simulink model "MPC_Quad"  (R2022b)
settings: Solver=FixedStepAuto  StartTime=0.0  StopTime=T_total  FixedStep=Ts  RelTol=1e-3
undefined symbols (not defined in the file): Alt_D, Alt_I, Alt_P, Att_Ang_P, Att_AngVel_D, Att_AngVel_I, Att_AngVel_P, Cm, Ct, DiscIntNeverNeededParam, estim_hover_nrpm, g, Ir, Ixx, Iyy, Izz, Length, mass, Pos_Pos_P, Pos_Vel_I, Pos_Vel_P, SampleTime, Yaw_D, Yaw_I, Yaw_P
libraries: slpidlib x4, simulink x2, mpclib x1
settings Model: PacingRate=0.350000  Creator=Bw Jiang  LastModifiedBy=Bw Jiang
settings DebuggingCC: AlgebraicLoopMsg=none  ParameterOverflowMsg=none  ParameterUnderflowMsg=error

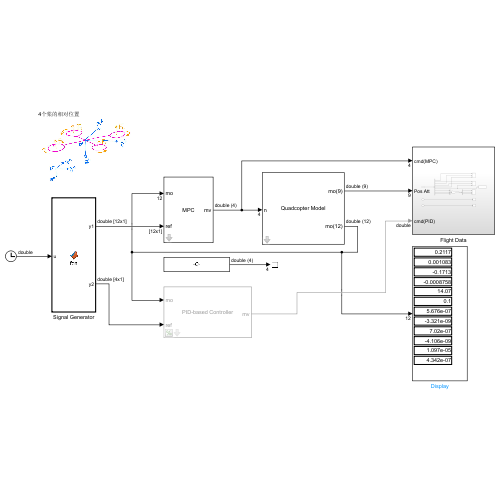
[thumbnail: Simulink's stored preview of the top-level diagram]
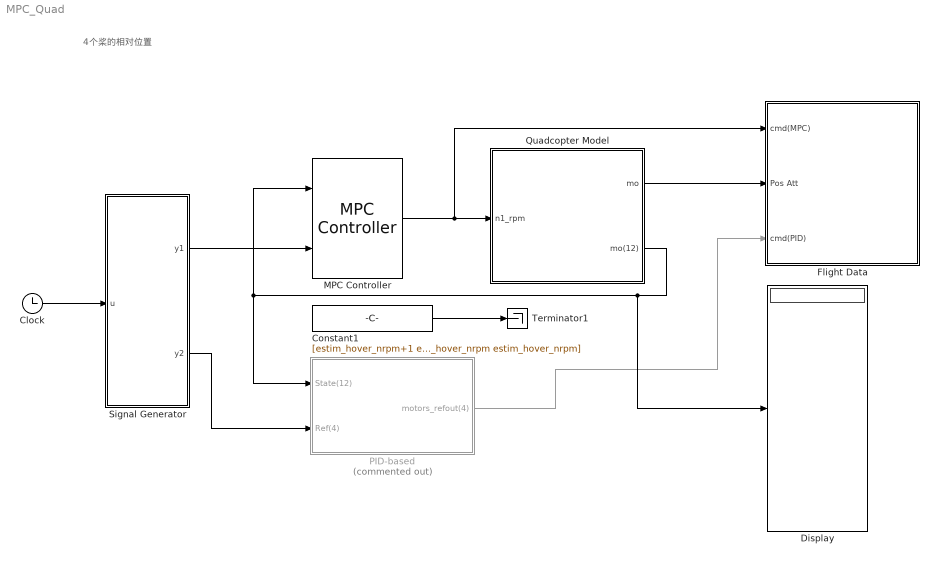
== system MPC_Quad ==
  note: 4个桨的相对位置
  Clock : Clock
  Constant1 : Constant  Value=[estim_hover_nrpm+1 estim_hover_nrpm estim_hover_nrpm estim_hover_nrpm]
  Display : Display
  Flight Data : Subsystem
  MPC Controller : mpclib/MPC Controller  SCDEnableBlockLinearizationSpecification=on  mpcobj=mpc1  is_multiple=0  enable_value=0  return_u0=off  updateMPCinCallerWorkspace=on  md_inport=off  mv_inport=off  uref_inport=off  return_cost=off  return_mvseq=off  return_qpstatus=off  return_xseq=off  return_state=off  return_ovseq=off  state_inport=off  umin_inport=off  umax_inport=off  ymin_inport=off  ymax_inport=off  cc_inport=off  ywt_inport=off  uwt_inport=off  duwt_inport=off  rhoeps_inport=off  pm_inport=off  MaximumP=10  HorizonChoice=FixedHorizon  n_ts=0.01  n_p=50  n_mv=4  n_md=0  n_ud=0  n_mo=12  n_uo=0  BlockDataType=double  SampleTimeInherited=off  switch_inport=off
  PID-based : Subsystem  Commented=on  mask{SampleTime=SampleTime, Pos_Pos_P=Pos_Pos_P, Pos_Vel_P=Pos_Vel_P, Pos_Vel_I=Pos_Vel_I, Alt_P=Alt_P, Alt_I=Alt_I, Alt_D=Alt_D, Yaw_P=Yaw_P, Yaw_I=Yaw_I, Yaw_D=Yaw_D, Att_Ang_P=Att_Ang_P, Att_AngVel_P=Att_AngVel_P, Att_AngVel_I=Att_AngVel_I, Att_AngVel_D=Att_AngVel_D}
      mask prompts: Pos_Pos_P "PosController.PositionLoop.P"; Pos_Vel_P "PosController.VelocityLoop.P"; Pos_Vel_I "PosController.VelocityLoop.I"; Alt_P "AltController.P"; Alt_I "AltController.I"; Alt_D "AltController.D"; Yaw_P "YawController.P"; Yaw_I "YawController.I"; Yaw_D "YawController.D"; Att_Ang_P "AttController.AngleLoop.P"; Att_AngVel_P "AttController.AngleVelocityLoop.P"; Att_AngVel_I "AttController.AngleVelocityLoop.I"; Att_AngVel_D "AttController.AngleVelocityLoop.D"
      mask init:
      | run("Scripts\PID_based_controller_init.m");
      mask DialogControl ParameterGroupVar Prompt: 参数
      mask Display:
      | disp('PID-based Controller');
      | port_label('output', 1, 'mv')
      | port_label('input', 1, 'mo')
      | port_label('input', 2, 'ref')
  Quadcopter Model : Subsystem  mask{g=g, mass=mass, I_xx=Ixx, I_yy=Iyy, I_zz=Izz, I_r=Ir, L=Length, C_M=Cm, C_T=Ct}
      mask prompts: g "Gravity"; I_xx "Inertia_xx"; I_yy "Inertia_yy"; I_zz "Inertia_zz"; I_r "Inertia_per_rotor"; L "Length"
      mask DialogControl ParameterGroupVar Prompt: 参数
      mask Display:
      | disp('Quadcopter Model');
      | port_label('input', 1, 'n')
      | % port_label('input', 2, 'n2')
      | % port_label('input', 3, 'n3')
      | % port_label('input', 4, 'n4')
      | port_label('output', 1, 'mo(9)')
      | port_label('output', 2, 'mo(12)')
      | % port_label('output', 3, 'y')
      | % port_label('output', 4, 'vy')
      | % port_label('output', 5, 'z')
      | % port_label('output', 6, 'vz')
      | % port_label('output', 7, 'phi')
      | % port_label('output', 8, 'd_phi')
      | % port_label('output', 9, 'theta')
      | % port_label('output', 10, 'd_theta')
      | % port_label('output', 11, 'psi')
      | % port_label('output', 12, 'd_psi')
  Signal Generator : MATLAB Function  TreatAsAtomicUnit=on
  Terminator1 : Terminator
  wires:
  Signal Generator/1(y1) -> MPC Controller/2
  Clock/1 -> Signal Generator/1(u)
  PID-based/1(motors_refout(4)) -> Flight Data/3(cmd(PID))
  MPC Controller/1 -> Quadcopter Model/1(n1_rpm), Flight Data/1(cmd(MPC))
  Signal Generator/2(y2) -> PID-based/2(Ref(4))
  Constant1/1 -> Terminator1/1
  Quadcopter Model/1(mo) -> Flight Data/2(Pos Att)
  Quadcopter Model/2(mo(12)) -> Display/1, MPC Controller/1, PID-based/1(State(12))

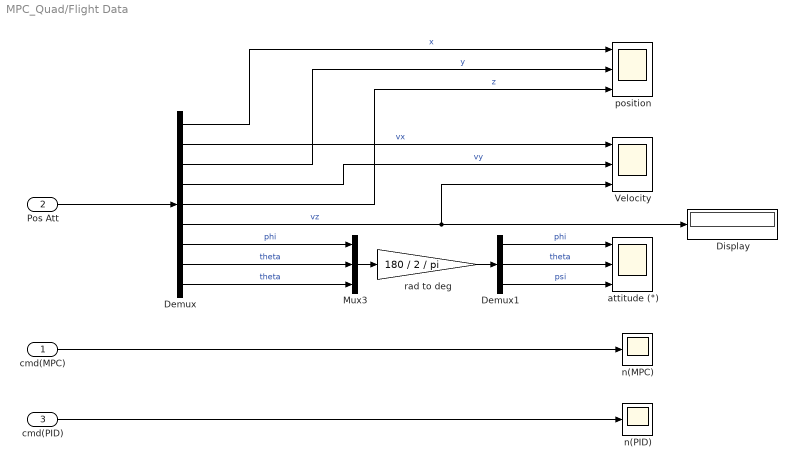
== system MPC_Quad/Flight Data ==
  cmd(MPC) : Inport
  Pos Att : Inport  Port=2
  cmd(PID) : Inport  Port=3
  Demux : Demux  Outputs=9
  Demux1 : Demux  Outputs=3
  Display : Display
  Mux3 : Mux  Inputs=3
  Velocity : Scope  NumInputPorts=3
  attitude (°) : Scope  NumInputPorts=3
  n(MPC) : Scope
  n(PID) : Scope
  position : Scope  NumInputPorts=3
  rad to deg : Gain  Gain=180 / 2 / pi
  wires:
  Demux/8 -> Mux3/2  "theta"
  Demux/4 -> Velocity/2  "vy"
  Demux/2 -> Velocity/1  "vx"
  Demux/7 -> Mux3/1  "phi"
  Demux/6 -> Velocity/3, Display/1  "vz"
  cmd(PID)/1 -> n(PID)/1
  Demux/5 -> position/3  "z"
  Demux/1 -> position/1  "x"
  Demux1/1 -> attitude (°)/1  "phi"
  Demux/3 -> position/2  "y"
  Demux1/2 -> attitude (°)/2  "theta"
  rad to deg/1 -> Demux1/1
  Demux1/3 -> attitude (°)/3  "psi"
  Mux3/1 -> rad to deg/1
  cmd(MPC)/1 -> n(MPC)/1
  Pos Att/1 -> Demux/1
  Demux/9 -> Mux3/3  "theta"

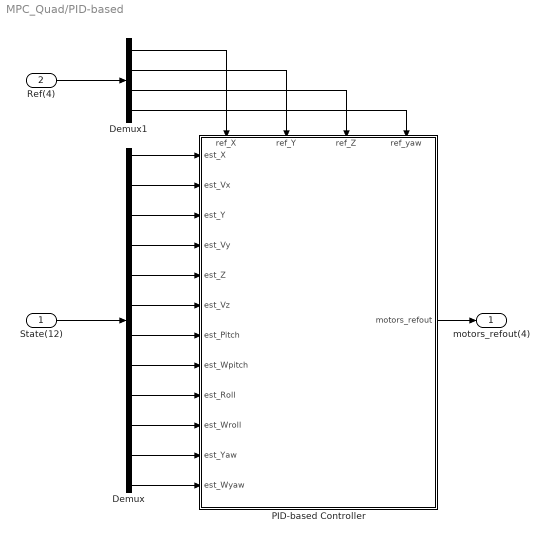
== system MPC_Quad/PID-based ==
  State(12) : Inport
  Ref(4) : Inport  Port=2
  Demux : Demux  Outputs=12
  Demux1 : Demux
  PID-based Controller : Subsystem
      settings: PortSchema="{\"entries\":[{\"content\":{\"sides\":[{\"content\":{\"connectorIds\":[\"In1\",\"In2\",\"In3\",\"In4\",\"In5\",\"In6\",\"In7\",\"In8\",\"In9\",\"In10\",\"In11\",\"In12\"]},\"type\":\"ConnectorPlacement.EquallySpacedRectSide\",\"uuid\":\"809a58d1-8f24-4346-a9a1-bdf3f40071a9\"},{\"content\":{\"connectorIds\":[\"Out1\"],\"side\":\"RIGHT\"},\"type\":\"ConnectorPlacement.EquallySpacedRectSide\",\"uuid\":\"e36db7a5-8644-49ff-9b48-8e381d81be19\"},{\"content\":{\"connectorIds\":[\"In13\",\"In14\",\"In15\",\"In16\"],\"side\":\"TOP\"},\"type\":\"ConnectorPlacement.EquallySpacedRectSide\",\"uuid\":\"d8c211b6-7652-4be5-9d63-16c6c31a5cb3\"}]},\"type\":\"ConnectorPlacement.EquallySpacedConnector\",\"uuid\":\"28a38415-8484-4982-8141-ea2d794bbc37\"}],\"packageUris\":[\"http://schema.mathworks.com/mf0/Connector/R2020b\"],\"version\":\"1.0\"}"
  motors_refout(4) : Outport
  wires:
  State(12)/1 -> Demux/1
  Demux1/1 -> PID-based Controller/13(ref_X)
  Demux1/2 -> PID-based Controller/14(ref_Y)
  Demux/5 -> PID-based Controller/5(est_Z)
  Demux/6 -> PID-based Controller/6(est_Vz)
  Demux/12 -> PID-based Controller/12(est_Wyaw)
  Demux/2 -> PID-based Controller/2(est_Vx)
  Demux1/3 -> PID-based Controller/15(ref_Z)
  Demux/11 -> PID-based Controller/11(est_Yaw)
  Demux/1 -> PID-based Controller/1(est_X)
  Demux/3 -> PID-based Controller/3(est_Y)
  Demux/4 -> PID-based Controller/4(est_Vy)
  Demux1/4 -> PID-based Controller/16(ref_yaw)
  PID-based Controller/1(motors_refout) -> motors_refout(4)/1
  Ref(4)/1 -> Demux1/1
  Demux/7 -> PID-based Controller/7(est_Pitch)
  Demux/8 -> PID-based Controller/8(est_Wpitch)
  Demux/9 -> PID-based Controller/9(est_Roll)
  Demux/10 -> PID-based Controller/10(est_Wroll)

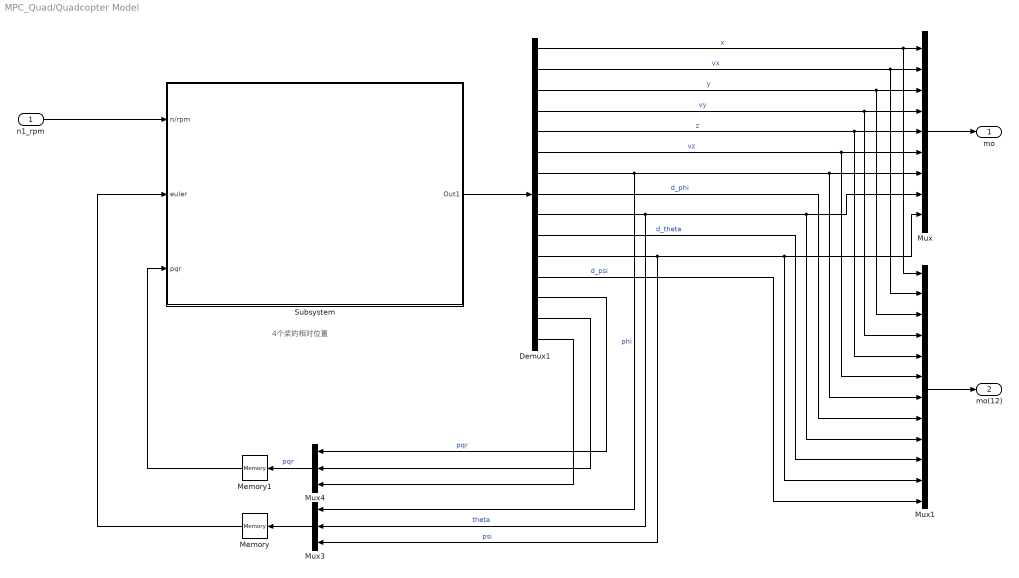
== system MPC_Quad/Quadcopter Model ==
  note: 4个桨的相对位置
  n1_rpm : Inport
  Demux1 : Demux  Outputs=15
  Memory : Memory  InheritSampleTime=on
  Memory1 : Memory  InheritSampleTime=on
  Mux : Mux  Inputs=9
  Mux1 : Mux  Inputs=12
  Mux3 : Mux  Inputs=3
  Mux4 : Mux  Inputs=3
  Subsystem : Subsystem
  mo : Outport
  mo(12) : Outport  Port=2
  wires:
  n1_rpm/1 -> Subsystem/1(n/rpm)
  Mux/1 -> mo/1
  Mux1/1 -> mo(12)/1
  Memory1/1 -> Subsystem/3(pqr)
  Demux1/15 -> Mux4/3
  Demux1/8 -> Mux1/8  "d_phi"
  Demux1/13 -> Mux4/1  "pqr"
  Mux4/1 -> Memory1/1  "pqr"
  Demux1/9 -> Mux/8, Mux1/9, Mux3/2  "theta"
  Demux1/10 -> Mux1/10  "d_theta"
  Demux1/1 -> Mux1/1, Mux/1  "x"
  Demux1/2 -> Mux/2, Mux1/2  "vx"
  Demux1/11 -> Mux/9, Mux1/11, Mux3/3  "psi"
  Demux1/4 -> Mux/4, Mux1/4  "vy"
  Demux1/3 -> Mux/3, Mux1/3  "y"
  Demux1/5 -> Mux/5, Mux1/5  "z"
  Subsystem/1(Out1) -> Demux1/1
  Demux1/12 -> Mux1/12  "d_psi"
  Memory/1 -> Subsystem/2(euler)
  Demux1/6 -> Mux/6, Mux1/6  "vz"
  Demux1/7 -> Mux/7, Mux1/7, Mux3/1  "phi"
  Mux3/1 -> Memory/1
  Demux1/14 -> Mux4/2

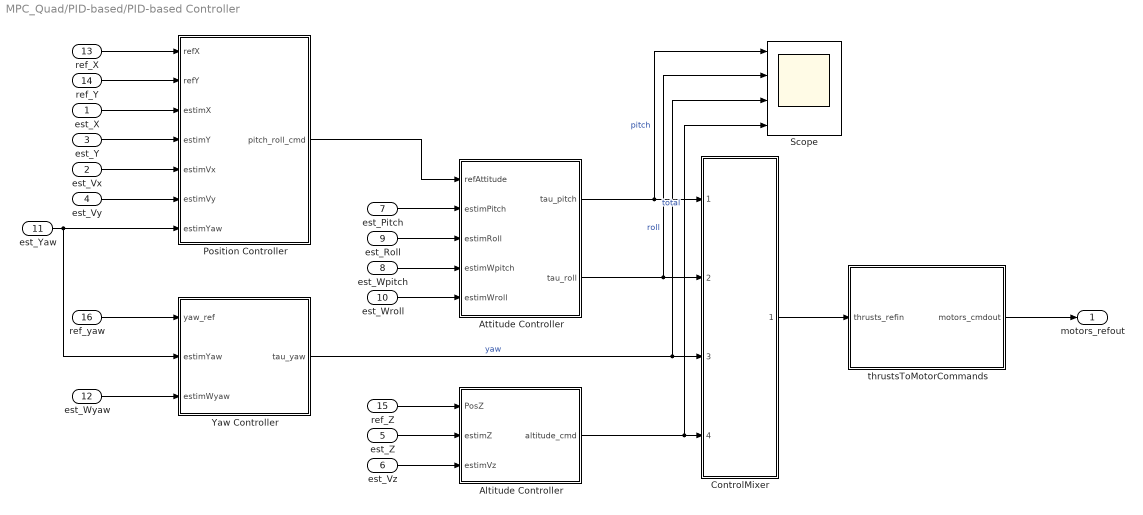
== system MPC_Quad/PID-based/PID-based Controller ==
  est_X : Inport
  est_Vx : Inport  Port=2
  est_Y : Inport  Port=3
  est_Vy : Inport  Port=4
  est_Z : Inport  Port=5
  est_Vz : Inport  Port=6
  est_Pitch : Inport  Port=7
  est_Wpitch : Inport  Port=8
  est_Roll : Inport  Port=9
  est_Wroll : Inport  Port=10
  est_Yaw : Inport  Port=11
  est_Wyaw : Inport  Port=12
  ref_X : Inport  Port=13
  ref_Y : Inport  Port=14
  ref_Z : Inport  Port=15
  ref_yaw : Inport  Port=16
  Altitude Controller : Subsystem
  Attitude Controller : Subsystem
  ControlMixer : Subsystem
  Position Controller : Subsystem
  Scope : Scope  NumInputPorts=4
  Yaw Controller : Subsystem
  thrustsToMotorCommands : Subsystem
  motors_refout : Outport  VectorParamsAs1DForOutWhenUnconnected=off
  wires:
  ControlMixer/1(thrusts_refout) -> thrustsToMotorCommands/1(thrusts_refin)
  est_X/1 -> Position Controller/3(estimX)
  est_Pitch/1 -> Attitude Controller/2(estimPitch)
  est_Vz/1 -> Altitude Controller/3(estimVz)
  ref_X/1 -> Position Controller/1(refX)
  est_Z/1 -> Altitude Controller/2(estimZ)
  Attitude Controller/1(tau_pitch) -> ControlMixer/1(tau_pitch), Scope/1  "pitch"
  ref_yaw/1 -> Yaw Controller/1(yaw_ref)
  est_Y/1 -> Position Controller/4(estimY)
  ref_Z/1 -> Altitude Controller/1(PosZ)
  Position Controller/1(pitch_roll_cmd) -> Attitude Controller/1(refAttitude)
  est_Wroll/1 -> Attitude Controller/5(estimWroll)
  ref_Y/1 -> Position Controller/2(refY)
  Attitude Controller/2(tau_roll) -> ControlMixer/2(tau_roll), Scope/2  "roll"
  est_Vx/1 -> Position Controller/5(estimVx)
  est_Wyaw/1 -> Yaw Controller/3(estimWyaw)
  Altitude Controller/1(altitude_cmd) -> Scope/4, ControlMixer/4(totalThrust)  "total"
  est_Yaw/1 -> Position Controller/7(estimYaw), Yaw Controller/2(estimYaw)
  est_Wpitch/1 -> Attitude Controller/4(estimWpitch)
  Yaw Controller/1(tau_yaw) -> ControlMixer/3(tau_yaw), Scope/3  "yaw"
  est_Vy/1 -> Position Controller/6(estimVy)
  thrustsToMotorCommands/1(motors_cmdout) -> motors_refout/1
  est_Roll/1 -> Attitude Controller/3(estimRoll)

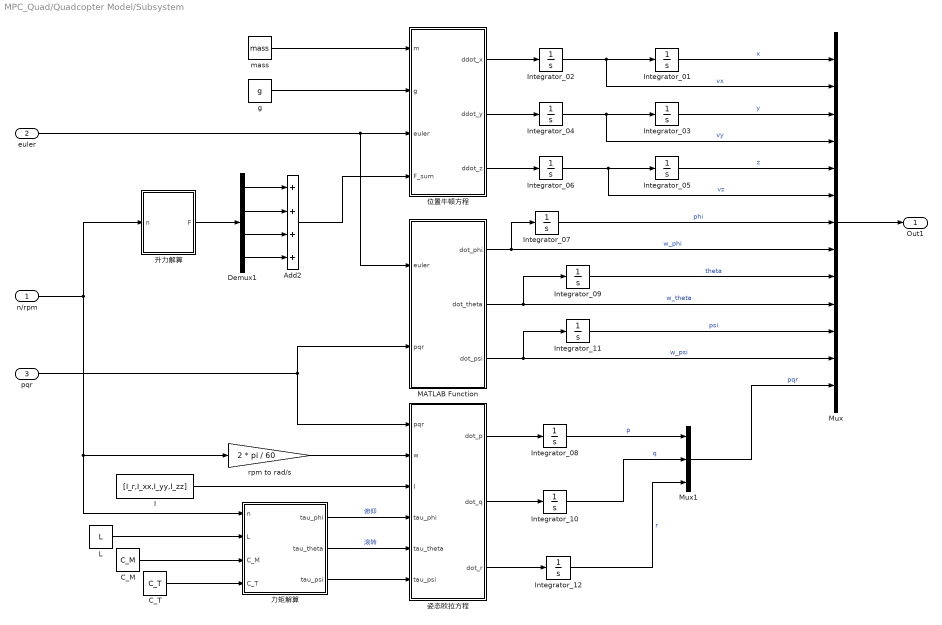
== system MPC_Quad/Quadcopter Model/Subsystem ==
  n/rpm : Inport  PortDimensions=4
  euler : Inport  Port=2  PortDimensions=3
  pqr : Inport  Port=3  PortDimensions=3
  Add2 : Sum  Inputs=++++
  C_M : Constant  Value=C_M
  C_T : Constant  Value=C_T
  Demux1 : Demux
  I : Constant  Value=[I_r,I_xx,I_yy,I_zz]
  Integrator_01 : Integrator
  Integrator_02 : Integrator
  Integrator_03 : Integrator
  Integrator_04 : Integrator
  Integrator_05 : Integrator
  Integrator_06 : Integrator
  Integrator_07 : Integrator
  Integrator_08 : Integrator
  Integrator_09 : Integrator
  Integrator_10 : Integrator
  Integrator_11 : Integrator
  Integrator_12 : Integrator
  L : Constant  Value=L
  MATLAB Function : MATLAB Function  TreatAsAtomicUnit=on
  Mux : Mux  Inputs=13
  Mux1 : Mux  Inputs=3
  g : Constant  Value=g
  mass : Constant  Value=mass
  rpm to rad/s : Gain  Gain=2 * pi / 60
  位置牛顿方程 : MATLAB Function  TreatAsAtomicUnit=on
  力矩解算 : MATLAB Function  TreatAsAtomicUnit=on
  升力解算 : MATLAB Function  TreatAsAtomicUnit=on
  姿态欧拉方程 : MATLAB Function  TreatAsAtomicUnit=on
  Out1 : Outport
  wires:
  姿态欧拉方程/1(dot_p) -> Integrator_08/1
  Demux1/4 -> Add2/4
  pqr/1 -> MATLAB Function/2(pqr), 姿态欧拉方程/1(pqr)
  位置牛顿方程/2(ddot_y) -> Integrator_04/1
  姿态欧拉方程/2(dot_q) -> Integrator_10/1
  I/1 -> 姿态欧拉方程/3(I)
  位置牛顿方程/3(ddot_z) -> Integrator_06/1
  Mux/1 -> Out1/1
  g/1 -> 位置牛顿方程/2(g)
  位置牛顿方程/1(ddot_x) -> Integrator_02/1
  Integrator_10/1 -> Mux1/2  "q"
  Demux1/1 -> Add2/1
  力矩解算/1(tau_phi) -> 姿态欧拉方程/4(tau_phi)  "俯仰"
  Integrator_08/1 -> Mux1/1  "p"
  euler/1 -> MATLAB Function/1(euler), 位置牛顿方程/3(euler)
  Integrator_03/1 -> Mux/3  "y"
  Integrator_09/1 -> Mux/9  "theta"
  力矩解算/3(tau_psi) -> 姿态欧拉方程/6(tau_psi)
  Demux1/2 -> Add2/2
  Add2/1 -> 位置牛顿方程/4(F_sum)
  Integrator_12/1 -> Mux1/3  "r"
  mass/1 -> 位置牛顿方程/1(m)
  力矩解算/2(tau_theta) -> 姿态欧拉方程/5(tau_theta)  "滚转"
  Demux1/3 -> Add2/3
  Integrator_05/1 -> Mux/5  "z"
  Integrator_01/1 -> Mux/1  "x"
  Integrator_02/1 -> Integrator_01/1, Mux/2  "vx"
  Integrator_07/1 -> Mux/7  "phi"
  Integrator_04/1 -> Mux/4, Integrator_03/1  "vy"
  Integrator_06/1 -> Mux/6, Integrator_05/1  "vz"
  Integrator_11/1 -> Mux/11  "psi"
  姿态欧拉方程/3(dot_r) -> Integrator_12/1
  MATLAB Function/3(dot_psi) -> Integrator_11/1, Mux/12  "w_psi"
  MATLAB Function/2(dot_theta) -> Integrator_09/1, Mux/10  "w_theta"
  MATLAB Function/1(dot_phi) -> Integrator_07/1, Mux/8  "w_phi"
  Mux1/1 -> Mux/13  "pqr"
  升力解算/1(F) -> Demux1/1
  L/1 -> 力矩解算/2(L)
  n/rpm/1 -> 升力解算/1(n), rpm to rad/s/1, 力矩解算/1(n)
  rpm to rad/s/1 -> 姿态欧拉方程/2(w)
  C_M/1 -> 力矩解算/3(C_M)
  C_T/1 -> 力矩解算/4(C_T)

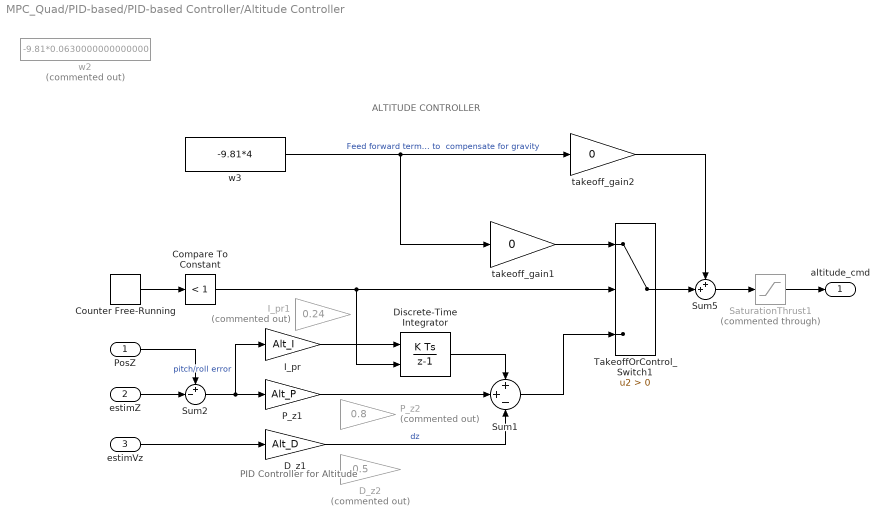
== system MPC_Quad/PID-based/PID-based Controller/Altitude Controller ==
  note: PID Controller for Altitude
  note: ALTITUDE CONTROLLER
  PosZ : Inport
  estimZ : Inport  Port=2
  estimVz : Inport  Port=3
  Compare To Constant : simulink/Logic and Bit Operations/Compare To Constant  relop=<  const=1  OutDataTypeStr=boolean
  Counter Free-Running : simulink/Sources/Counter Free-Running  NumBits=16  tsamp=-1
  D_z1 : Gain  Gain=Alt_D  SaturateOnIntegerOverflow=on
  D_z2 : Gain  Commented=on  Gain=0.5  ParamDataTypeStr=single  OutDataTypeStr=single  SaturateOnIntegerOverflow=on
  Discrete-Time Integrator : DiscreteIntegrator  ExternalReset=falling  SampleTime=SampleTime  LimitOutput=on  UpperSaturationLimit=2  LowerSaturationLimit=-2  ICPrevOutput=DiscIntNeverNeededParam  ICPrevScaledInput=DiscIntNeverNeededParam
  I_pr : Gain  Gain=Alt_I
  I_pr1 : Gain  Commented=on  Gain=0.24
  P_z1 : Gain  Gain=Alt_P  SaturateOnIntegerOverflow=on
  P_z2 : Gain  Commented=on  Gain=0.8  ParamDataTypeStr=single  OutDataTypeStr=single  SaturateOnIntegerOverflow=on
  SaturationThrust1 : Saturate  Commented=through  UpperLimit=4*0.920000000000000*0.326642213351703  LowerLimit=-4*0.920000000000000*0.326642213351703
  Sum1 : Sum  Inputs=++-  SaturateOnIntegerOverflow=on
  Sum2 : Sum  Inputs=+-|  SaturateOnIntegerOverflow=on
  Sum5 : Sum  Inputs=++|  AccumDataTypeStr=double  OutDataTypeStr=double  SaturateOnIntegerOverflow=on
  TakeoffOrControl_Switch1 : Switch  Criteria=u2 > Threshold  SaturateOnIntegerOverflow=off  InputSameDT=off
  takeoff_gain1 : Gain  Gain=0  ParamDataTypeStr=single  OutDataTypeStr=double  SaturateOnIntegerOverflow=on
  takeoff_gain2 : Gain  Gain=0  ParamDataTypeStr=single  OutDataTypeStr=double  SaturateOnIntegerOverflow=on
  w2 : Constant  Commented=on  Value=-9.81*0.0630000000000000  OutDataTypeStr=double  SampleTime=0.005
  w3 : Constant  Value=-9.81*4  VectorParams1D=off  OutDataTypeStr=double  SampleTime=0.005
  altitude_cmd : Outport  VectorParamsAs1DForOutWhenUnconnected=off
  wires:
  TakeoffOrControl_Switch1/1 -> Sum5/2
  Discrete-Time Integrator/1 -> Sum1/1
  PosZ/1 -> Sum2/1
  P_z1/1 -> Sum1/2
  Counter Free-Running/1 -> Compare To Constant/1
  estimVz/1 -> D_z1/1
  Sum5/1 -> SaturationThrust1/1
  estimZ/1 -> Sum2/2
  D_z1/1 -> Sum1/3  "dz"
  Sum1/1 -> TakeoffOrControl_Switch1/3
  takeoff_gain1/1 -> TakeoffOrControl_Switch1/1
  Sum2/1 -> I_pr/1, P_z1/1  "pitch/roll error"
  I_pr/1 -> Discrete-Time Integrator/1
  SaturationThrust1/1 -> altitude_cmd/1
  Compare To Constant/1 -> Discrete-Time Integrator/2, TakeoffOrControl_Switch1/2
  w3/1 -> takeoff_gain1/1, takeoff_gain2/1  "Feed forward term to  compensate for gravity"
  takeoff_gain2/1 -> Sum5/1

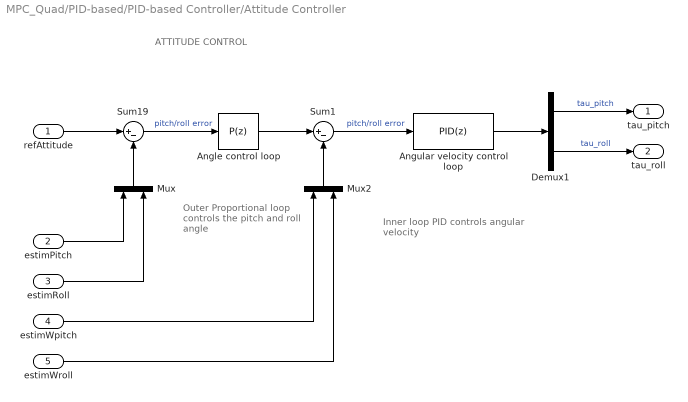
== system MPC_Quad/PID-based/PID-based Controller/Attitude Controller ==
  note: Inner loop PID
      | controls angular velocity
  note: Outer Proportional loop
      | controls the pitch and roll angle
  note: ATTITUDE CONTROL
  refAttitude : Inport
  estimPitch : Inport  Port=2
  estimRoll : Inport  Port=3
  estimWpitch : Inport  Port=4
  estimWroll : Inport  Port=5
  Angle control loop : slpidlib/PID Controller  Controller=P  Form=Parallel  TimeDomain=Discrete-time  UseExternalTs=off  SampleTime=SampleTime  IntegratorMethod=Forward Euler  FilterMethod=Forward Euler  ControllerParametersSource=internal  P=Att_Ang_P  I=1  UseKiTs=off  D=0  N=100  UseFilter=on  TunerSelectOption=Transfer Function Based (PID Tuner App)  InitialConditionSource=internal  InitialConditionForIntegrator=0  InitialConditionForFilter=0  DifferentiatorICPrevScaledInput=0  ExternalReset=none  TrackingMode=off  Kt=1  LimitOutput=off  SatLimitsSource=internal  UpperSaturationLimit=inf  LowerSaturationLimit=-inf  LinearizeAsGain=on  AntiWindupMode=none  Kb=1  LimitIntegrator=off  UpperIntegratorSaturationLimit=inf  LowerIntegratorSaturationLimit=-inf  POutMin=[]  POutMax=[]  IOutMin=[]  IOutMax=[]  DOutMin=[]  DOutMax=[]  NOutMin=[]  NOutMax=[]  SumOutMin=[]  SumOutMax=[]  SaturationOutMin=[]  SaturationOutMax=[]  PParamMin=[]  PParamMax=[]  IParamMin=[]  IParamMax=[]  DParamMin=[]  DParamMax=[]  NParamMin=[]  NParamMax=[]  KbParamMin=[]  KbParamMax=[]  KtParamMin=[]  KtParamMax=[]  KbOutMin=[]  KbOutMax=[]  KtOutMin=[]  KtOutMax=[]  IntegratorOutMin=[]  IntegratorOutMax=[]  FilterOutMin=[]  FilterOutMax=[]  SumI1OutMin=[]  SumI1OutMax=[]  SumI2OutMin=[]  SumI2OutMax=[]  SumI3OutMin=[]  SumI3OutMax=[]  SumI4OutMin=[]  SumI4OutMax=[]  SumDOutMin=[]  SumDOutMax=[]  DifferentiatorOutMin=[]  DifferentiatorOutMax=[]  FilterDiffOutCoefMin=[]  FilterDiffOutCoefMax=[]  ReciprocalOutMin=[]  ReciprocalOutMax=[]  SumDenOutMin=[]  SumDenOutMax=[]  SumNumOutMin=[]  SumNumOutMax=[]  DivideOutMin=[]  DivideOutMax=[]  UdiffTsProdOutMin=[]  UdiffTsProdOutMax=[]  NTsProdOutMin=[]  NTsProdOutMax=[]  UintegralTsProdOutMin=[]  UintegralTsProdOutMax=[]  UngainTsProdOutMin=[]  UngainTsProdOutMax=[]  ClampingZeroOutDataTypeStr=Inherit: Inherit via back propagation  ClampingZeroOutMin=[]  ClampingZeroOutMax=[]  FilterDenConstantOutDataTypeStr=Inherit: Inherit via back propagation  FilterDenConstantOutMin=[]  FilterDenConstantOutMax=[]  PCopyOutDataTypeStr=Inherit: Inherit via back propagation  PCopyOutMin=[]  PCopyOutMax=[]  NCopyOutDataTypeStr=Inherit: Inherit via back propagation  NCopyOutMin=[]  NCopyOutMax=[]  IntegratorContinuousStateAttributes=''  IntegratorStateMustResolveToSignalObject=off  IntegratorRTWStateStorageClass=Auto  FilterContinuousStateAttributes=''  FilterStateMustResolveToSignalObject=off  FilterRTWStateStorageClass=Auto  ParallelPVariant=InternalParameters  IdealPVariant=Disabled  IVariant=Disabled  DVariant=Disabled  IntegratorVariant=Disabled  SatVariant=Disabled  AWVariant=Disabled  PCopyVariant=Disabled  TRVariant=Disabled  FdbkBlocksVariant=Forward  IdealPFdbkVariant=Disabled  SatFdbkVariant=Disabled  DerivativeFilterVariant=Disabled  NVariant=Disabled  NCopyVariant=Disabled_SignalSpec  FilterICVariant=Disabled  IntegratorICVariant=Disabled  ExternalResetVariant=Disabled  TRSumVariant=Passthrough  SumFdbkVariant=Disabled  SumVariant=Passthrough_P  TsampFilterVariant=InternalTs  TsampNgainVariant=Passthrough  TsampIntegralVariant=Disabled_SignalSpec  ExternalSaturationOutDataTypeStr=Inherit: Same as second input
  Angular velocity control loop : slpidlib/PID Controller  Controller=PID  Form=Parallel  TimeDomain=Discrete-time  UseExternalTs=off  SampleTime=SampleTime  IntegratorMethod=Forward Euler  FilterMethod=Forward Euler  ControllerParametersSource=internal  P=Att_AngVel_P  I=Att_AngVel_I  UseKiTs=off  D=Att_AngVel_D  N=70*[1 1]  UseFilter=on  TunerSelectOption=Transfer Function Based (PID Tuner App)  InitialConditionSource=internal  InitialConditionForIntegrator=0  InitialConditionForFilter=0  DifferentiatorICPrevScaledInput=0  ExternalReset=none  TrackingMode=off  Kt=1  LimitOutput=on  SatLimitsSource=internal  UpperSaturationLimit=0.02  LowerSaturationLimit=-0.02  LinearizeAsGain=on  AntiWindupMode=clamping  Kb=1  LimitIntegrator=off  UpperIntegratorSaturationLimit=inf  LowerIntegratorSaturationLimit=-inf  PGainOutDataTypeStr=double  PProdOutDataTypeStr=double  POutMin=[]  POutMax=[]  IGainOutDataTypeStr=double  IProdOutDataTypeStr=double  IOutMin=[]  IOutMax=[]  DGainOutDataTypeStr=double  DProdOutDataTypeStr=double  DOutMin=[]  DOutMax=[]  NGainOutDataTypeStr=double  NProdOutDataTypeStr=double  NOutMin=[]  NOutMax=[]  SumOutDataTypeStr=double  SumOutMin=[]  SumOutMax=[]  SaturationOutDataTypeStr=double  SaturationOutMin=[]  SaturationOutMax=[]  PParamMin=[]  PParamMax=[]  IParamMin=[]  IParamMax=[]  DParamMin=[]  DParamMax=[]  NParamMin=[]  NParamMax=[]  KbParamMin=[]  KbParamMax=[]  KtParamMin=[]  KtParamMax=[]  KbOutMin=[]  KbOutMax=[]  KtOutMin=[]  KtOutMax=[]  IntegratorOutMin=[]  IntegratorOutMax=[]  FilterOutMin=[]  FilterOutMax=[]  SumI1OutMin=[]  SumI1OutMax=[]  SumI2OutMin=[]  SumI2OutMax=[]  SumI3OutMin=[]  SumI3OutMax=[]  SumI4OutMin=[]  SumI4OutMax=[]  SumDOutMin=[]  SumDOutMax=[]  DifferentiatorOutMin=[]  DifferentiatorOutMax=[]  FilterDiffOutCoefMin=[]  FilterDiffOutCoefMax=[]  ReciprocalOutMin=[]  ReciprocalOutMax=[]  SumDenOutMin=[]  SumDenOutMax=[]  SumNumOutMin=[]  SumNumOutMax=[]  DivideOutMin=[]  DivideOutMax=[]  UdiffTsProdOutMin=[]  UdiffTsProdOutMax=[]  NTsProdOutMin=[]  NTsProdOutMax=[]  UintegralTsProdOutMin=[]  UintegralTsProdOutMax=[]  UngainTsProdOutMin=[]  UngainTsProdOutMax=[]  ClampingZeroOutDataTypeStr=Inherit: Inherit via back propagation  ClampingZeroOutMin=[]  ClampingZeroOutMax=[]  FilterDenConstantOutDataTypeStr=Inherit: Inherit via back propagation  FilterDenConstantOutMin=[]  FilterDenConstantOutMax=[]  PCopyOutDataTypeStr=Inherit: Inherit via back propagation  PCopyOutMin=[]  PCopyOutMax=[]  NCopyOutDataTypeStr=Inherit: Inherit via back propagation  NCopyOutMin=[]  NCopyOutMax=[]  IntegratorContinuousStateAttributes=''  IntegratorStateMustResolveToSignalObject=off  IntegratorRTWStateStorageClass=Auto  FilterContinuousStateAttributes=''  FilterStateMustResolveToSignalObject=off  FilterRTWStateStorageClass=Auto  ParallelPVariant=InternalParameters  IdealPVariant=Disabled  IVariant=InternalParameters  DVariant=InternalParameters  IntegratorVariant=Discrete  SatVariant=Enabled  AWVariant=DiscClampingParallel  PCopyVariant=Disabled  TRVariant=Disabled  FdbkBlocksVariant=Forward  IdealPFdbkVariant=Disabled  SatFdbkVariant=Disabled  DerivativeFilterVariant=ForwardEulerFilter  NVariant=InternalParameters  NCopyVariant=Disabled  FilterICVariant=InternalICsFilter  IntegratorICVariant=InternalICs  ExternalResetVariant=Disabled  TRSumVariant=Passthrough  SumFdbkVariant=Disabled  SumVariant=Sum_PID  TsampFilterVariant=InternalTs  TsampNgainVariant=Passthrough  TsampIntegralVariant=Passthrough  ExternalSaturationOutDataTypeStr=Inherit: Same as second input
  Demux1 : Demux  Outputs=2
  Mux : Mux  Inputs=2
  Mux2 : Mux  Inputs=2
  Sum1 : Sum  Inputs=|+-
  Sum19 : Sum  Inputs=|+-
  tau_pitch : Outport  VectorParamsAs1DForOutWhenUnconnected=off
  tau_roll : Outport  Port=2  OutDataTypeStr=double  VectorParamsAs1DForOutWhenUnconnected=off
  wires:
  Sum1/1 -> Angular velocity control loop/1  "pitch/roll error"
  Angle control loop/1 -> Sum1/1
  Mux2/1 -> Sum1/2
  Sum19/1 -> Angle control loop/1  "pitch/roll error"
  Angular velocity control loop/1 -> Demux1/1
  Demux1/2 -> tau_roll/1  "tau_roll"
  Demux1/1 -> tau_pitch/1  "tau_pitch"
  Mux/1 -> Sum19/2
  refAttitude/1 -> Sum19/1
  estimPitch/1 -> Mux/1
  estimRoll/1 -> Mux/2
  estimWpitch/1 -> Mux2/1
  estimWroll/1 -> Mux2/2

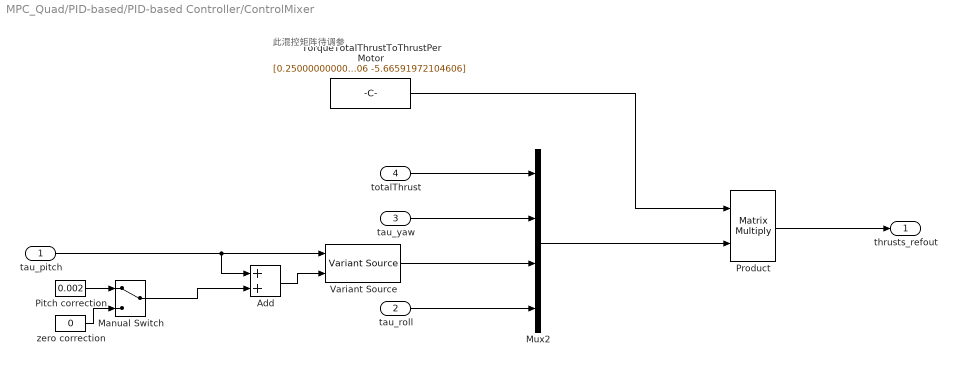
== system MPC_Quad/PID-based/PID-based Controller/ControlMixer ==
  note: 此混控矩阵待调参
  tau_pitch : Inport
  tau_roll : Inport  Port=2
  tau_yaw : Inport  Port=3
  totalThrust : Inport  Port=4  OutDataTypeStr=double
  Add : Sum
  Manual Switch : ManualSwitch
  Mux2 : Mux
  Pitch correction : Constant  Value=0.002
  Product : Product  Multiplication=Matrix(*)  RndMeth=Zero
  TorqueTotalThrustToThrustPerMotor : Constant  Value="[0.250000000000000\t103.573625306767\t-5.66591972104605\t-5.66591972104606; 0.250000000000000\t-103.573625306767\t-5.66591972104606\t5.66591972104606; 0.250000000000000\t103.573625306767\t5.66591972104606\t5.66591972104606; 0.250000000000000\t-103.573625306767\t5.66591972104606\t-5.66591972104606]"  OutDataTypeStr=double  SampleTime=SampleTime
  Variant Source : VariantSource  VariantControlMode=sim codegen switching  VariantActivationTime=update diagram analyze all choices  ShowConditionOnBlock=on
  zero correction : Constant  Value=0
  thrusts_refout : Outport  VectorParamsAs1DForOutWhenUnconnected=off
  wires:
  Product/1 -> thrusts_refout/1
  tau_roll/1 -> Mux2/4
  Add/1 -> Variant Source/2
  totalThrust/1 -> Mux2/1
  TorqueTotalThrustToThrustPerMotor/1 -> Product/1
  Mux2/1 -> Product/2
  Variant Source/1 -> Mux2/3
  tau_pitch/1 -> Add/1, Variant Source/1
  Pitch correction/1 -> Manual Switch/1
  zero correction/1 -> Manual Switch/2
  Manual Switch/1 -> Add/2
  tau_yaw/1 -> Mux2/2

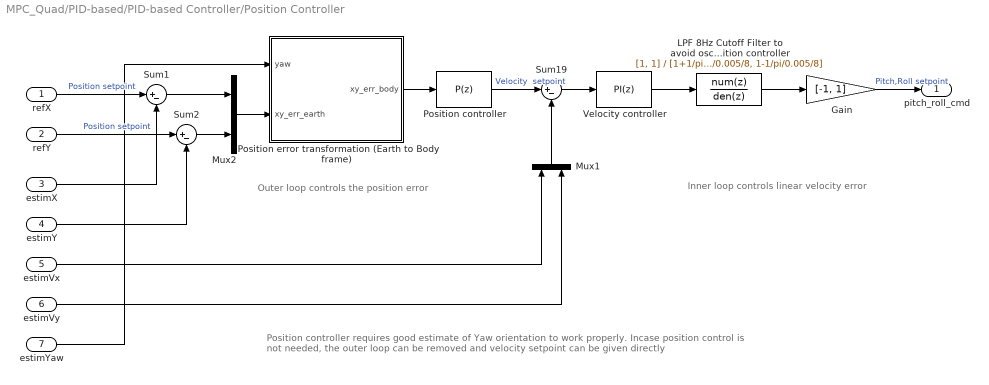
== system MPC_Quad/PID-based/PID-based Controller/Position Controller ==
  note: Position controller requires good estimate of Yaw orientation to work properly.
      | Incase position control is not needed, the outer loop can be removed and velocity setpoint can be given directly
  note: Inner loop controls linear velocity error
  note: Outer loop controls the position error
  refX : Inport
  refY : Inport  Port=2
  estimX : Inport  Port=3
  estimY : Inport  Port=4
  estimVx : Inport  Port=5
  estimVy : Inport  Port=6
  estimYaw : Inport  Port=7
  Gain : Gain  Gain=[-1, 1]
  LPF 8Hz Cutoff Filter to avoid oscillations induced by position controller : DiscreteTransferFcn  Numerator=[1, 1]  Denominator=[1+1/pi/0.005/8, 1-1/pi/0.005/8]
  Mux1 : Mux  Inputs=2
  Mux2 : Mux  Inputs=2
  Position controller : slpidlib/PID Controller  Controller=P  Form=Parallel  TimeDomain=Discrete-time  UseExternalTs=off  SampleTime=SampleTime  IntegratorMethod=Forward Euler  FilterMethod=Forward Euler  ControllerParametersSource=internal  P=Pos_Pos_P  I=0.1  UseKiTs=off  D=0  N=100  UseFilter=on  TunerSelectOption=Transfer Function Based (PID Tuner App)  InitialConditionSource=internal  InitialConditionForIntegrator=0  InitialConditionForFilter=0  DifferentiatorICPrevScaledInput=0  ExternalReset=none  TrackingMode=off  Kt=1  LimitOutput=on  SatLimitsSource=internal  UpperSaturationLimit=0.5  LowerSaturationLimit=-0.5  LinearizeAsGain=on  AntiWindupMode=clamping  Kb=1  LimitIntegrator=off  UpperIntegratorSaturationLimit=inf  LowerIntegratorSaturationLimit=-inf  POutMin=[]  POutMax=[]  IOutMin=[]  IOutMax=[]  DOutMin=[]  DOutMax=[]  NOutMin=[]  NOutMax=[]  SumOutMin=[]  SumOutMax=[]  SaturationOutMin=[]  SaturationOutMax=[]  PParamMin=[]  PParamMax=[]  IParamMin=[]  IParamMax=[]  DParamMin=[]  DParamMax=[]  NParamMin=[]  NParamMax=[]  KbParamMin=[]  KbParamMax=[]  KtParamMin=[]  KtParamMax=[]  KbOutMin=[]  KbOutMax=[]  KtOutMin=[]  KtOutMax=[]  IntegratorOutMin=[]  IntegratorOutMax=[]  FilterOutMin=[]  FilterOutMax=[]  SumI1OutMin=[]  SumI1OutMax=[]  SumI2OutMin=[]  SumI2OutMax=[]  SumI3OutMin=[]  SumI3OutMax=[]  SumI4OutMin=[]  SumI4OutMax=[]  SumDOutMin=[]  SumDOutMax=[]  DifferentiatorOutMin=[]  DifferentiatorOutMax=[]  FilterDiffOutCoefMin=[]  FilterDiffOutCoefMax=[]  ReciprocalOutMin=[]  ReciprocalOutMax=[]  SumDenOutMin=[]  SumDenOutMax=[]  SumNumOutMin=[]  SumNumOutMax=[]  DivideOutMin=[]  DivideOutMax=[]  UdiffTsProdOutMin=[]  UdiffTsProdOutMax=[]  NTsProdOutMin=[]  NTsProdOutMax=[]  UintegralTsProdOutMin=[]  UintegralTsProdOutMax=[]  UngainTsProdOutMin=[]  UngainTsProdOutMax=[]  ClampingZeroOutDataTypeStr=Inherit: Inherit via back propagation  ClampingZeroOutMin=[]  ClampingZeroOutMax=[]  FilterDenConstantOutDataTypeStr=Inherit: Inherit via back propagation  FilterDenConstantOutMin=[]  FilterDenConstantOutMax=[]  PCopyOutDataTypeStr=Inherit: Inherit via back propagation  PCopyOutMin=[]  PCopyOutMax=[]  NCopyOutDataTypeStr=Inherit: Inherit via back propagation  NCopyOutMin=[]  NCopyOutMax=[]  IntegratorContinuousStateAttributes=''  IntegratorStateMustResolveToSignalObject=off  IntegratorRTWStateStorageClass=Auto  FilterContinuousStateAttributes=''  FilterStateMustResolveToSignalObject=off  FilterRTWStateStorageClass=Auto  ParallelPVariant=InternalParameters  IdealPVariant=Disabled  IVariant=Disabled  DVariant=Disabled  IntegratorVariant=Disabled  SatVariant=Enabled  AWVariant=Disabled  PCopyVariant=Disabled  TRVariant=Disabled  FdbkBlocksVariant=Forward  IdealPFdbkVariant=Disabled  SatFdbkVariant=Disabled  DerivativeFilterVariant=Disabled  NVariant=Disabled  NCopyVariant=Disabled_SignalSpec  FilterICVariant=Disabled  IntegratorICVariant=Disabled  ExternalResetVariant=Disabled  TRSumVariant=Passthrough  SumFdbkVariant=Disabled  SumVariant=Passthrough_P  TsampFilterVariant=InternalTs  TsampNgainVariant=Passthrough  TsampIntegralVariant=Disabled_SignalSpec  ExternalSaturationOutDataTypeStr=Inherit: Same as second input
  Position error transformation (Earth to Body frame) : MATLAB Function  TreatAsAtomicUnit=on
  Sum1 : Sum  Inputs=|+-
  Sum19 : Sum  Inputs=|+-
  Sum2 : Sum  Inputs=|+-
  Velocity controller : slpidlib/PID Controller  Controller=PI  Form=Parallel  TimeDomain=Discrete-time  UseExternalTs=off  SampleTime=SampleTime  IntegratorMethod=Forward Euler  FilterMethod=Forward Euler  ControllerParametersSource=internal  P=Pos_Vel_P  I=Pos_Vel_I  UseKiTs=off  D=0  N=100  UseFilter=on  TunerSelectOption=Transfer Function Based (PID Tuner App)  InitialConditionSource=internal  InitialConditionForIntegrator=0  InitialConditionForFilter=0  DifferentiatorICPrevScaledInput=0  ExternalReset=none  TrackingMode=off  Kt=1  LimitOutput=on  SatLimitsSource=internal  UpperSaturationLimit=20*pi/180  LowerSaturationLimit=-20*pi/180  LinearizeAsGain=on  AntiWindupMode=clamping  Kb=1  LimitIntegrator=off  UpperIntegratorSaturationLimit=inf  LowerIntegratorSaturationLimit=-inf  POutMin=[]  POutMax=[]  IOutMin=[]  IOutMax=[]  DOutMin=[]  DOutMax=[]  NOutMin=[]  NOutMax=[]  SumOutMin=[]  SumOutMax=[]  SaturationOutMin=[]  SaturationOutMax=[]  PParamMin=[]  PParamMax=[]  IParamMin=[]  IParamMax=[]  DParamMin=[]  DParamMax=[]  NParamMin=[]  NParamMax=[]  KbParamMin=[]  KbParamMax=[]  KtParamMin=[]  KtParamMax=[]  KbOutMin=[]  KbOutMax=[]  KtOutMin=[]  KtOutMax=[]  IntegratorOutMin=[]  IntegratorOutMax=[]  FilterOutMin=[]  FilterOutMax=[]  SumI1OutMin=[]  SumI1OutMax=[]  SumI2OutMin=[]  SumI2OutMax=[]  SumI3OutMin=[]  SumI3OutMax=[]  SumI4OutMin=[]  SumI4OutMax=[]  SumDOutMin=[]  SumDOutMax=[]  DifferentiatorOutMin=[]  DifferentiatorOutMax=[]  FilterDiffOutCoefMin=[]  FilterDiffOutCoefMax=[]  ReciprocalOutMin=[]  ReciprocalOutMax=[]  SumDenOutMin=[]  SumDenOutMax=[]  SumNumOutMin=[]  SumNumOutMax=[]  DivideOutMin=[]  DivideOutMax=[]  UdiffTsProdOutMin=[]  UdiffTsProdOutMax=[]  NTsProdOutMin=[]  NTsProdOutMax=[]  UintegralTsProdOutMin=[]  UintegralTsProdOutMax=[]  UngainTsProdOutMin=[]  UngainTsProdOutMax=[]  ClampingZeroOutDataTypeStr=Inherit: Inherit via back propagation  ClampingZeroOutMin=[]  ClampingZeroOutMax=[]  FilterDenConstantOutDataTypeStr=Inherit: Inherit via back propagation  FilterDenConstantOutMin=[]  FilterDenConstantOutMax=[]  PCopyOutDataTypeStr=Inherit: Inherit via back propagation  PCopyOutMin=[]  PCopyOutMax=[]  NCopyOutDataTypeStr=Inherit: Inherit via back propagation  NCopyOutMin=[]  NCopyOutMax=[]  IntegratorContinuousStateAttributes=''  IntegratorStateMustResolveToSignalObject=off  IntegratorRTWStateStorageClass=Auto  FilterContinuousStateAttributes=''  FilterStateMustResolveToSignalObject=off  FilterRTWStateStorageClass=Auto  ParallelPVariant=InternalParameters  IdealPVariant=Disabled  IVariant=InternalParameters  DVariant=Disabled  IntegratorVariant=Discrete  SatVariant=Enabled  AWVariant=DiscClampingParallel  PCopyVariant=Disabled  TRVariant=Disabled  FdbkBlocksVariant=Forward  IdealPFdbkVariant=Disabled  SatFdbkVariant=Disabled  DerivativeFilterVariant=Disabled  NVariant=Disabled  NCopyVariant=Disabled_SignalSpec  FilterICVariant=Disabled  IntegratorICVariant=InternalICs  ExternalResetVariant=Disabled  TRSumVariant=Passthrough  SumFdbkVariant=Disabled  SumVariant=Sum_PI  TsampFilterVariant=InternalTs  TsampNgainVariant=Passthrough  TsampIntegralVariant=Passthrough  ExternalSaturationOutDataTypeStr=Inherit: Same as second input
  pitch_roll_cmd : Outport  VectorParamsAs1DForOutWhenUnconnected=off
  wires:
  estimVx/1 -> Mux1/1
  estimY/1 -> Sum2/2
  estimVy/1 -> Mux1/2
  Mux1/1 -> Sum19/2
  Sum19/1 -> Velocity controller/1
  Velocity controller/1 -> LPF 8Hz Cutoff Filter to avoid oscillations induced by position controller/1
  Gain/1 -> pitch_roll_cmd/1  "Pitch,Roll setpoint"
  LPF 8Hz Cutoff Filter to avoid oscillations induced by position controller/1 -> Gain/1
  Position controller/1 -> Sum19/1  "Velocity  setpoint"
  Position error transformation (Earth to Body frame)/1(xy_err_body) -> Position controller/1
  refX/1 -> Sum1/1  "Position setpoint"
  Sum1/1 -> Mux2/1
  Mux2/1 -> Position error transformation (Earth to Body frame)/2(xy_err_earth)
  refY/1 -> Sum2/1  "Position setpoint"
  Sum2/1 -> Mux2/2
  estimX/1 -> Sum1/2
  estimYaw/1 -> Position error transformation (Earth to Body frame)/1(yaw)

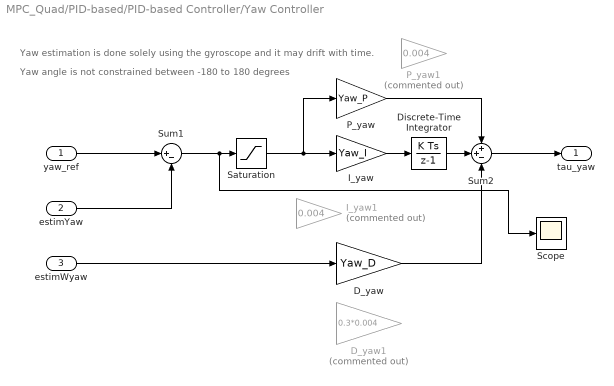
== system MPC_Quad/PID-based/PID-based Controller/Yaw Controller ==
  note: Yaw angle is not constrained between -180 to 180 degrees
  note: Yaw estimation is done solely using the gyroscope and it may drift with time.
  yaw_ref : Inport
  estimYaw : Inport  Port=2
  estimWyaw : Inport  Port=3
  D_yaw : Gain  Gain=Yaw_D
  D_yaw1 : Gain  Commented=on  Gain=0.3*0.004
  Discrete-Time Integrator : DiscreteIntegrator  gainval=1  SampleTime=-1  ICPrevOutput=DiscIntNeverNeededParam  ICPrevScaledInput=DiscIntNeverNeededParam
  I_yaw : Gain  Gain=Yaw_I
  I_yaw1 : Gain  Commented=on  Gain=0.004  ParamDataTypeStr=single  OutDataTypeStr=single
  P_yaw : Gain  Gain=Yaw_P
  P_yaw1 : Gain  Commented=on  Gain=0.004  ParamDataTypeStr=single  OutDataTypeStr=single
  Saturation : Saturate  UpperLimit=pi/180*30  LowerLimit=-pi/180*30
  Scope : Scope
  Sum1 : Sum  Inputs=|+-  SaturateOnIntegerOverflow=on
  Sum2 : Sum  Inputs=++-
  tau_yaw : Outport  VectorParamsAs1DForOutWhenUnconnected=off
  wires:
  D_yaw/1 -> Sum2/3
  P_yaw/1 -> Sum2/1
  Sum1/1 -> Scope/1, Saturation/1
  estimYaw/1 -> Sum1/2
  yaw_ref/1 -> Sum1/1
  Sum2/1 -> tau_yaw/1
  Discrete-Time Integrator/1 -> Sum2/2
  I_yaw/1 -> Discrete-Time Integrator/1
  Saturation/1 -> P_yaw/1, I_yaw/1
  estimWyaw/1 -> D_yaw/1

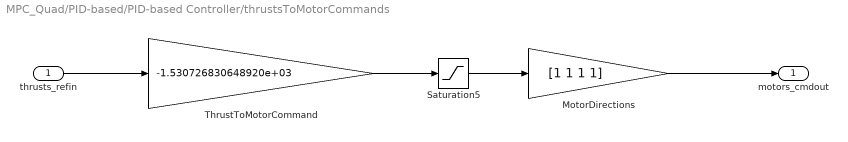
== system MPC_Quad/PID-based/PID-based Controller/thrustsToMotorCommands ==
  thrusts_refin : Inport
  MotorDirections : Gain  Gain=[1 1 1 1]
  Saturation5 : Saturate  UpperLimit=10000  LowerLimit=1000
  ThrustToMotorCommand : Gain  Gain=-1.530726830648920e+03
  motors_cmdout : Outport  VectorParamsAs1DForOutWhenUnconnected=off
  wires:
  Saturation5/1 -> MotorDirections/1
  MotorDirections/1 -> motors_cmdout/1
  ThrustToMotorCommand/1 -> Saturation5/1
  thrusts_refin/1 -> ThrustToMotorCommand/1

== matlab function MPC_Quad/Quadcopter Model/Subsystem/MATLAB Function ==
  data: euler input; pqr input; dot_phi output; dot_theta output; dot_psi output
function [dot_phi, dot_theta, dot_psi] = fcn(euler, pqr)

% 角加速度的坐标转换，从机体系b到惯性系e

p = pqr(1);
q = pqr(2);
r = pqr(3);

phi =euler(1);
theta = euler(2);
psi = euler(3);

mat = [
    1, tan(theta) * sin(phi), tan(theta) * cos(phi);
    0, cos(phi), -sin(phi);
    0, sin(phi) / cos(theta), cos(phi) / cos(theta)
    ];
body = [p; q; r];
earth = mat * body;

dot_phi = earth(1);
dot_theta = earth(2);
dot_psi = earth(3);

== matlab function MPC_Quad/Quadcopter Model/Subsystem/位置牛顿方程 ==
  data: m input; g input; euler input; ddot_x output; F_sum input; ddot_y output; ddot_z output
function [ddot_x, ddot_y, ddot_z] = fcn(m, g, euler, F_sum)

% F_sum恒正

phi =euler(1);
theta = euler(2);
psi = euler(3);

ddot_x = -(cos(phi) * sin(theta) * cos(psi) + sin(phi) * sin(psi)) * F_sum / m;
ddot_y = -(cos(phi) * sin(theta) * sin(psi) - sin(phi) * cos(psi)) * F_sum / m;
ddot_z = -cos(phi) * cos(theta) * F_sum / m + g;

end

== matlab function MPC_Quad/Quadcopter Model/Subsystem/姿态欧拉方程 ==
  data: pqr input; dot_p output; w input; I input; dot_q output; dot_r output; tau_phi input; tau_theta input; tau_psi input
function [dot_p, dot_q, dot_r] = fcn(pqr, w, I, tau_phi, tau_theta, tau_psi)

w1 = w(1);
w2 = w(2);
w3 = w(3);
w4 = w(4);

p = pqr(1);
q = pqr(2);
r = pqr(3);

I_r = I(1);
I_xx = I(2);
I_yy = I(3);
I_zz = I(4);

w_tau = w1 - w2 + w3 - w4;

dot_p = (I_yy - I_zz) / I_xx * q * r - I_r * q / I_xx * w_tau + tau_phi / I_xx;
dot_q = (I_zz - I_xx) / I_yy * p * r + I_r * p / I_yy * w_tau + tau_theta / I_yy;
dot_r = (I_xx - I_yy) / I_zz * q * p + tau_psi / I_zz;

end

== matlab function MPC_Quad/Quadcopter Model/Subsystem/升力解算 ==
  data: n input; F output
function F = fcn(n)
%% Input Vars
% n - rpm

%% Output Vars
% F - N

%% Mid Vars
% omega - rad/s

%% Code

% F = n .* n * 2.414e-7 * 2;

omega = n / 60 * 2 * pi;
F = omega .* omega * 1.11e-5;

end

== matlab function MPC_Quad/Signal Generator ==
  data: u input; y1 output; y2 output
function [y1, y2] = fcn(u)

y1 = u * [0.1
          0 
          0 
          0 
          0
          0
          0
          0
          0 
          0 
          0 
          0];

y2 = [0
      0 
      0 
      0];

end

== matlab function MPC_Quad/Quadcopter Model/Subsystem/力矩解算 ==
  data: n input; L input; tau_phi output; tau_theta output; tau_psi output; C_M input; C_T input
function [tau_phi, tau_theta, tau_psi]= fcn(n, L, C_M, C_T)
%% Input Vars
% n - rpm
% L - m
% C_M - N*m*s^2/rad^2
% C_T - N*s^2/rad^2

%% Output Vars
% tau - N*m

%% Mid Vars
% w - rad/s

%% Code

% C_T = 1.1e-5;
% C_M = 1.0144e-7;

% F1 = F(1);
% F2 = F(2);
% F3 = F(3);
% F4 = F(4);

w1 = n(1) / 60 * 2 * pi;
w2 = n(2) / 60 * 2 * pi;
w3 = n(3) / 60 * 2 * pi;
w4 = n(4) / 60 * 2 * pi;

% I_r = I(1);

% w_tau = w1 + w3 - w2 - w4;

% 横滚
tau_phi = sqrt(2) / 2 * C_T * L * (w1^2 - w2^2 - w3^2 + w4^2); % tau_phi = (F1+F2-F3-F4) * L;
% 俯仰
tau_theta = sqrt(2) / 2 * C_T * L * (w1^2 + w2^2 - w3^2 - w4^2); % tau_theta = (F1-F2-F3+F4) * L;
% 偏航
tau_psi = C_M * (w1^2 - w2^2 + w3^2 - w4^2); % tau_psi = w_tau * I_r;

end

== matlab function MPC_Quad/PID-based/PID-based Controller/Position Controller/Position error transformation (Earth to Body frame) ==
  data: yaw input; xy_err_earth input; xy_err_body output
function xy_err_body = fcn(yaw,xy_err_earth)

transformation = [cos(yaw), sin(yaw); -sin(yaw),  cos(yaw)];
xy_err_body = transformation * xy_err_earth;


end
